simulink model "example_WorkingTime"  (R2018b)
settings: Solver=ode45  StartTime=0.0  StopTime=30  MaxStep=0.1  RelTol=1e-3  EnableMultiTasking=on
libraries: carnot x1
settings Model: Creator=drhf  LastModifiedBy=drhf
settings DataIOCC: LimitDataPoints=on  SaveFormat=Array
settings OptimizationCC: DefaultParameterBehavior=Inlined  LifeSpan=inf
settings DebuggingCC: UnderspecifiedInitializationDetection=Classic  MergeDetectMultiDrivingBlocksExec=none  SolverPrmCheckMsg=warning  SFUnexpectedBacktrackingDiag=warning  SFNoUnconditionalDefaultTransitionDiag=warning  SFExecutionAtInitializationDiag=none
settings HardwareCC: ProdBitPerPointer=32  ProdBitPerSizeT=32  ProdBitPerPtrDiffT=32  ProdLargestAtomicFloat=None  ProdIntDivRoundTo=Undefined  ProdEndianess=Unspecified  ProdWordSize=32  ProdHWDeviceType=32-bit Generic
settings ModelReferenceCC: PropagateSignalLabelsOutOfModel=off
settings SFSimCC: SimUseLocalCustomCode=off
settings RTWCC: RTWUseLocalCustomCode=off
settings CodeAppCC: StateflowObjectComments=on
settings GRTTargetCC: TargetLangStandard=C89/C90 (ANSI)  GeneratePreprocessorConditionals=Disable all
settings ConfigComp: CovMetricSettings=dw  CovHtmlReporting=on  CovSaveCumulativeToWorkspaceVar=on  CovSaveSingleToWorkspaceVar=on  CovExternalEMLEnable=off

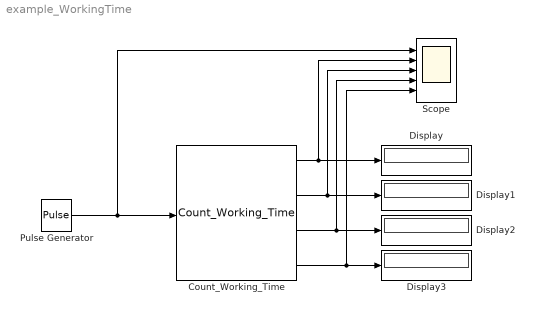
== system example_WorkingTime ==
  Count_Working_Time : carnot/Toolbox/Count_Working_Time
  Display{,1..3} (4 alike) : Display
  Pulse Generator : DiscretePulseGenerator  PulseType=Time based  Period=10  PulseWidth=10  PhaseDelay=1
  Scope : Scope  NumInputPorts=5
  wires:
  Pulse Generator/1 -> Scope/1, Count_Working_Time/1
  Count_Working_Time/1 -> Display/1, Scope/2
  Count_Working_Time/2 -> Scope/3, Display1/1
  Count_Working_Time/3 -> Scope/4, Display2/1
  Count_Working_Time/4 -> Scope/5, Display3/1
